simulink library "Power_Components_4Battery"  (R2018b)
settings: Solver=VariableStepAuto  StartTime=0.0  StopTime=10.0  RelTol=1e-3
undefined symbols (not defined in the file or in its folder): B1, B2, B3, B4, Power
libraries: fl_lib x7, nesl_utility x7, elec_lib x6, simulink_extras x1
Description:
  | Component of Simscape Vehicle Templates Library
  | 
  | Copyright 2018-2020 The MathWorks, Inc.
settings Model: Creator=smiller  LastModifiedBy=smiller

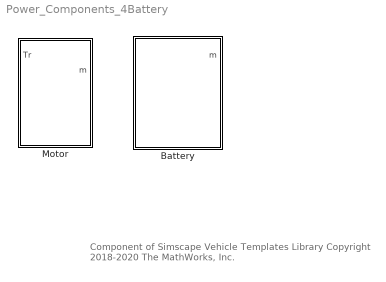
== system Power_Components_4Battery ==
  note: Component of Simscape Vehicle Templates Library
      | Copyright 2018-2020 The MathWorks, Inc.
  Battery : Subsystem
      mask Display: image('sm_car_vehicle_power_battery_system_IMAGE.png');
  Motor : Subsystem  mask{Motor=Power.MotorRL}
      mask prompts: Motor "Motor (Structure)"
      mask Display: image('sm_car_vehicle_power_emotor_simplified_IMAGE.png');

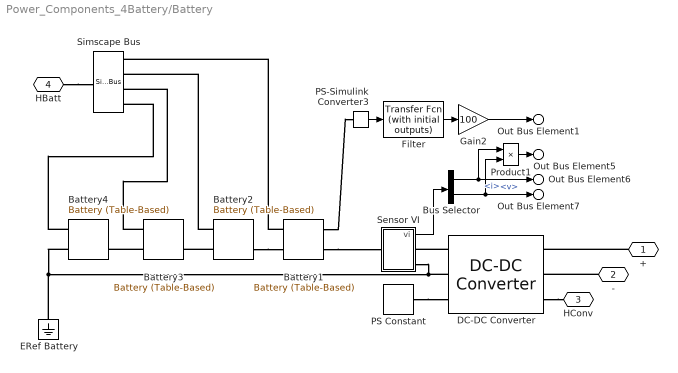
== system Power_Components_4Battery/Battery ==
  Battery{1..4} (4 alike) : elec_lib/Sources/Battery (Table-Based)  SOC_vec=Power.Battery.vNoLoad.SOC.Value  T_vec=Power.Battery.vNoLoad.T.Value K  V0_mat=Power.Battery.vNoLoad.V0.Value/4 V  R0_mat=Power.Battery.rTerminal.R0.Value/4 Ohm  AH_vec=Power.Battery.AhTable.Ah.Value/4 hr*A  prm_leak=1  Rleak_vec=[8000, 7000, 6000] Ohm  prm_dyn=1  R1_mat=[.089, .076, .01; .042, .022, .099; .019, .007, .002; .051, .043, .029] Ohm  tau1_mat=[44, 148, 235; 93, 110, 1000; 19, 27, 133; .5, 22, 3] s  R2_mat=[.014, .382, .407; .028, .006, .007; .014, .007, .006; .333, .956, .912] Ohm  tau2_mat=[1, 44, 5644; 11, 24, 506; 2, 14, 330; 3310, 13419, 30216] s  R3_mat=[.014, .382, .407; .028, .006, .007; .014, .007, .006; .333, .956, .912] Ohm  tau3_mat=[1, 44, 5644; 11, 24, 506; 2, 14, 330; 3310, 13419, 30216] s  R4_mat=[.014, .382, .407; .028, .006, .007; .014, .007, .006; .333, .956, .912] Ohm  tau4_mat=[1, 44, 5644; 11, 24, 506; 2, 14, 330; 3310, 13419, 30216] s  R5_mat=[.014, .382, .407; .028, .006, .007; .014, .007, .006; .333, .956, .912] Ohm  tau5_mat=[1, 44, 5644; 11, 24, 506; 2, 14, 330; 3310, 13419, 30216] s  N0=100  dV0=0  dR0=0  dAH=0  dRleak=0  dR1=0  dR2=0  dR3=0  dR4=0  dR5=0  temperature=300 K  i_specify=off  i_priority=None  i=0 A  i_nominal_specify=off  i_nominal_unit=A  i_nominal_value=1  v_specify=off  v_priority=None  v=0 V  v_nominal_specify=off  v_nominal_unit=V  v_nominal_value=1  stateOfCharge_specify=on  stateOfCharge_priority=High  stateOfCharge=Power.Battery.SOCInit.Value  stateOfCharge_nominal_specify=off  stateOfCharge_nominal_unit=1  stateOfCharge_nominal_value=1  num_cycles_specify=off  num_cycles_priority=High  num_cycles=0  num_cycles_nominal_specify=off  num_cycles_nominal_unit=1  num_cycles_nominal_value=1  thermal_mass=30000/4 J/K  temperature_specify=on  temperature_priority=High  temperature_nominal_specify=off  temperature_nominal_unit=K  temperature_nominal_value=1
      settings: SourceProductName=Simscape Electronics  SourceProductBaseCode=SN
  Bus Selector : BusSelector  OutputSignals=i,v
  DC-DC Converter : elec_lib/Sources/DC-DC Converter  v_ref=Power.Converter.vRef.Value V  P_rated=Power.Converter.Power.Value W  droop_param=1  droop=0.001*0 V/A  droop_percent=2  reversible=1  efficiency=Power.Converter.efficiency.Value  P_fixed=1 W  model_dynamics=1  tau=Power.Converter.fConverter.Value s  v_ini=Power.Converter.vRef.Value V  G_diode=1e-8 1/Ohm  i1_max=Power.Converter.iMaxSupply.Value A  fault_condition=1  fault_threshold=0.5  thermal_mass=500 J/K  initial_temperature=25 degC
      settings: SourceProductName=Simscape Electronics  SourceProductBaseCode=SN
  ERef Battery : fl_lib/Electrical/Electrical Elements/Electrical Reference
  Filter : simulink_extras/Additional Linear/Transfer Fcn (with initial outputs)  N=[1]  D=[.01 1]  Y0=Power.Battery.SOCInit.Value  U0=0
  Gain2 : Gain  Gain=100
  PS Constant : fl_lib/Physical Signals/Sources/PS Constant  constant=0
  PS-Simulink Converter3 : nesl_utility/PS-Simulink Converter  PhysicalDomain=network_engine_domain  SubClassName=ps_output  LeftPortType=input  RightPortType=output  PseudoPeriodic=off  Frequencies=[]  Unit=1  AffineConversion=off
      settings: SourceProductBaseCode=PW,SS
  Product1 : Product
  Sensor VI : Subsystem
  Simscape Bus : SimscapeBus  HierarchyStrings=B1;B2;B3;B4
  + : PMIOPort  Side=Right
  - : PMIOPort  Port=2  Side=Right
  HConv : PMIOPort  Port=3  Side=Right
  HBatt : PMIOPort  Port=4  Side=Left
  Out Bus Element5 : Outport  VectorParamsAs1DForOutWhenUnconnected=on  PortName=m  Element=Power
  Out Bus Element6 : Outport  VectorParamsAs1DForOutWhenUnconnected=on  PortName=m  Element=i
  Out Bus Element7 : Outport  VectorParamsAs1DForOutWhenUnconnected=on  PortName=m  Element=v
  Out Bus Element1 : Outport  VectorParamsAs1DForOutWhenUnconnected=on  PortName=m  Element=SOC
  wires:
  Sensor VI/1(vi) -> Bus Selector/1
  Bus Selector/2 -> Out Bus Element7/1, Product1/2  "<v>"
  Product1/1 -> Out Bus Element5/1
  Bus Selector/1 -> Product1/1, Out Bus Element6/1  "<i>"
  PS-Simulink Converter3/1 -> Filter/1
  Gain2/1 -> Out Bus Element1/1
  Filter/1 -> Gain2/1
  connections:
  DC-DC Converter/RConn3 -- HConv/RConn1
  -/RConn1 -- DC-DC Converter/RConn2
  Battery2/LConn1 -- Battery1/RConn1
  +/RConn1 -- DC-DC Converter/RConn1
  Battery1/LConn2 -- PS-Simulink Converter3/LConn1
  Battery1/RConn2 -- Simscape Bus/LConn1
  Battery1/LConn1 -- Sensor VI/LConn1
  DC-DC Converter/LConn1 -- Sensor VI/RConn1
  ERef Battery/LConn1 -- Battery4/RConn1 -- DC-DC Converter/LConn2 -- Sensor VI/RConn2
  Battery2/RConn1 -- Battery3/LConn1
  Battery3/RConn1 -- Battery4/LConn1
  HBatt/RConn1 -- Simscape Bus/RConn1
  Battery2/RConn2 -- Simscape Bus/LConn2
  Battery3/RConn2 -- Simscape Bus/LConn3
  Battery4/RConn2 -- Simscape Bus/LConn4
  PS Constant/RConn1 -- DC-DC Converter/LConn3

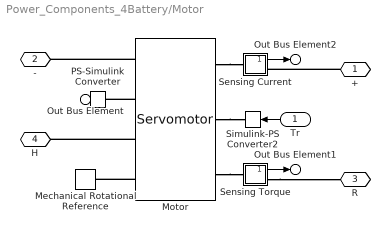
== system Power_Components_4Battery/Motor ==
  Tr : Inport
  Mechanical Rotational Reference : fl_lib/Mechanical/Rotational Elements/Mechanical Rotational Reference
  Motor : elec_lib/Actuators & Drivers/Rotational Actuators/Servomotor  torque_speed_param=1  w_t=Motor.TorqueSpd.w.Value rpm  T_t=Motor.TorqueSpd.trq.Value N*m  torque_max=0.1 N*m  power_max=30 W  Tc=1/Motor.fActuatorCutoff.Value s  losses_param=3  eff=100  w_eff=3750 rpm  T_eff=0.08 N*m  Piron=0 W  Pbase=0 W  w_eff_vec=Motor.LossTable.w.Value rpm  T_eff_vec=Motor.LossTable.trq.Value N*m  v_eff_vec=[100, 250, 400] V  losses_mat=[1.49, 1.67, 2.21, 3.1; .42, .69, 1.14, 2.03; .06, .24, .78, 1.68; .42, .69, 1.14, 2.03; 1.49, 1.67, 2.21, 3.1] W  efficiency_mat=Motor.LossTable.efficiency.Value  losses_mat_3D=ones(5, 4, 3) W  efficiency_mat_3D=95 * ones(5, 4, 3)  Res=0 Ohm  J=Motor.J.Value kg*m^2  lam=0 N*m/(rad/s)  speed0=0 rpm  faulted_specify=off  faulted_priority=None  faulted=0  faulted_nominal_specify=off  faulted_nominal_unit=1  faulted_nominal_value=1  alpha=3.93e-3 1/K  Tmeas=Motor.ThermalLoss.T1.Value degC  Tmeas2=Motor.ThermalLoss.T2.Value degC  losses_mat_T2=[1.49, 1.74, 2.49, 3.74; .42, .67, 1.42, 2.67; .06, .31, 1.06, 2.31; .42, .67, 1.42, 2.67; 1.49, 1.74, 2.49, 3.74] W  efficiency_mat_T2=Motor.ThermalLoss.efficiency.Value  losses_mat_3D_T2=ones(5, 4, 3) W  efficiency_mat_3D_T2=95 * ones(5, 4, 3)  thermal_mass=Motor.ThermalLoss.mThermal.Value J/K  initial_temperature=Motor.ThermalLoss.Tinit.Value K  fault_condition=1  fault_threshold=0.5
      settings: SourceProductName=Simscape Electronics  SourceProductBaseCode=SN
  PS-Simulink Converter : nesl_utility/PS-Simulink Converter  PhysicalDomain=network_engine_domain  SubClassName=ps_output  LeftPortType=input  RightPortType=output  PseudoPeriodic=off  Frequencies=[]  Unit=1  AffineConversion=off
      settings: SourceProductBaseCode=PW,SS
  Sensing Current : Subsystem
      mask Display: disp('i')
  Sensing Torque : Subsystem
      mask Display: disp('t');
  Simulink-PS Converter2 : nesl_utility/Simulink-PS Converter  PhysicalDomain=network_engine_domain  SubClassName=ps_input  LeftPortType=input  RightPortType=output  PseudoPeriodic=off  Frequencies=[]  NoiseDistribution=none  NoiseParameters=[]  Unit=N*m  AffineConversion=off  FilteringAndDerivatives=provide  SimscapeFilterOrder=1  InputFilterTimeConstant=0.001  UdotUserProvided=0
      settings: SourceProductBaseCode=PW,SS
  + : PMIOPort  Side=Left
  - : PMIOPort  Port=2  Side=Left
  R : PMIOPort  Port=3  Side=Right
  H : PMIOPort  Port=4  Side=Left
  Out Bus Element : Outport  PortName=m  Element=w
  Out Bus Element1 : Outport  PortName=m  Element=trq
  Out Bus Element2 : Outport  PortName=m  Element=i
  wires:
  PS-Simulink Converter/1 -> Out Bus Element/1
  Tr/1 -> Simulink-PS Converter2/1
  Sensing Current/1(Out1) -> Out Bus Element2/1
  Sensing Torque/1(T) -> Out Bus Element1/1
  connections:
  Motor/RConn2 -- PS-Simulink Converter/LConn1
  Motor/RConn4 -- Mechanical Rotational Reference/LConn1
  Motor/RConn3 -- H/RConn1
  Motor/LConn2 -- Simulink-PS Converter2/RConn1
  Motor/RConn1 -- -/RConn1
  Motor/LConn3 -- Sensing Torque/LConn1
  Sensing Torque/RConn1 -- R/RConn1
  +/RConn1 -- Sensing Current/RConn1
  Motor/LConn1 -- Sensing Current/LConn1

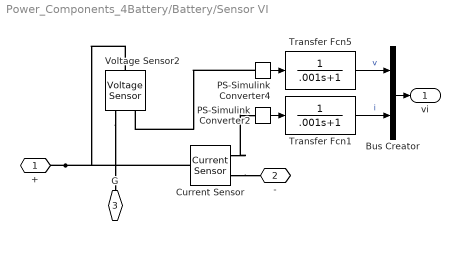
== system Power_Components_4Battery/Battery/Sensor VI ==
  Bus Creator : BusCreator  Inputs=2
  Current Sensor : fl_lib/Electrical/Electrical Sensors/Current Sensor
  PS-Simulink Converter2 : nesl_utility/PS-Simulink Converter  PhysicalDomain=network_engine_domain  SubClassName=ps_output  LeftPortType=input  RightPortType=output  PseudoPeriodic=off  Frequencies=[]  Unit=1  AffineConversion=off
      settings: SourceProductBaseCode=PW,SS
  PS-Simulink Converter4 : nesl_utility/PS-Simulink Converter  PhysicalDomain=network_engine_domain  SubClassName=ps_output  LeftPortType=input  RightPortType=output  PseudoPeriodic=off  Frequencies=[]  Unit=1  AffineConversion=off
      settings: SourceProductBaseCode=PW,SS
  Transfer Fcn1 : TransferFcn  Denominator=[.001 1]
  Transfer Fcn5 : TransferFcn  Denominator=[.001 1]
  Voltage Sensor2 : fl_lib/Electrical/Electrical Sensors/Voltage Sensor
  + : PMIOPort  Side=Left
  - : PMIOPort  Port=2  Side=Right
  G : PMIOPort  Port=3  Side=Right
  vi : Outport  VectorParamsAs1DForOutWhenUnconnected=on
  wires:
  PS-Simulink Converter4/1 -> Transfer Fcn5/1
  PS-Simulink Converter2/1 -> Transfer Fcn1/1
  Transfer Fcn1/1 -> Bus Creator/2  "i"
  Transfer Fcn5/1 -> Bus Creator/1  "v"
  Bus Creator/1 -> vi/1
  connections:
  +/RConn1 -- Current Sensor/LConn1 -- Voltage Sensor2/LConn1
  PS-Simulink Converter4/LConn1 -- Voltage Sensor2/RConn1
  Current Sensor/RConn2 -- -/RConn1
  Voltage Sensor2/RConn2 -- G/RConn1
  Current Sensor/RConn1 -- PS-Simulink Converter2/LConn1

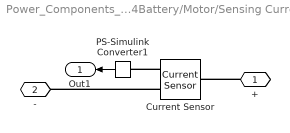
== system Power_Components_4Battery/Motor/Sensing Current ==
  Current Sensor : fl_lib/Electrical/Electrical Sensors/Current Sensor
  PS-Simulink Converter1 : nesl_utility/PS-Simulink Converter  PhysicalDomain=network_engine_domain  SubClassName=ps_output  LeftPortType=input  RightPortType=output  PseudoPeriodic=off  Frequencies=[]  Unit=1  AffineConversion=off
      settings: SourceProductBaseCode=PW,SS
  + : PMIOPort  Side=Right
  - : PMIOPort  Port=2  Side=Left
  Out1 : Outport
  wires:
  PS-Simulink Converter1/1 -> Out1/1
  connections:
  Current Sensor/RConn2 -- -/RConn1
  Current Sensor/RConn1 -- PS-Simulink Converter1/LConn1
  +/RConn1 -- Current Sensor/LConn1

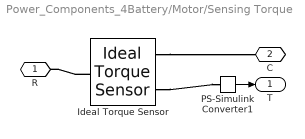
== system Power_Components_4Battery/Motor/Sensing Torque ==
  Ideal Torque Sensor : fl_lib/Mechanical/Mechanical Sensors/Ideal Torque Sensor
  PS-Simulink Converter1 : nesl_utility/PS-Simulink Converter  PhysicalDomain=network_engine_domain  SubClassName=ps_output  LeftPortType=input  RightPortType=output  PseudoPeriodic=off  Frequencies=[]  Unit=1  AffineConversion=off
      settings: SourceProductBaseCode=PW,SS
  R : PMIOPort  Side=Left
  C : PMIOPort  Port=2  Side=Right
  T : Outport
  wires:
  PS-Simulink Converter1/1 -> T/1
  connections:
  Ideal Torque Sensor/RConn2 -- PS-Simulink Converter1/LConn1
  Ideal Torque Sensor/RConn1 -- C/RConn1
  Ideal Torque Sensor/LConn1 -- R/RConn1
